simulink model "ev3_fix"  (R2018b)
settings: Solver=FixedStepAuto  StartTime=0.0  StopTime=10.0  RelTol=1e-3  EnableMultiTasking=on
libraries: legoev3lib x3
settings Model: ExtModeTrigDuration=2  Creator=chpark  LastModifiedBy=chpark
settings SolverCC: PositivePriorityOrder=on
settings OptimizationCC: EnhancedBackFolding=on  PassReuseOutputArgsAs=Individual arguments  MaxStackSize=64  OptimizeBlockOrder=speed  DifferentSizesBufferReuse=on  OptimizationCustomize=off
settings DebuggingCC: ParameterTunabilityLossMsg=error
settings HardwareCC: ProdBitPerPointer=32  ProdBitPerSizeT=32  ProdBitPerPtrDiffT=32  ProdLargestAtomicInteger=Long  ProdWordSize=32  ProdHWDeviceType=ARM Compatible->ARM 9  UseEmbeddedCoderFeatures=off  UseSimulinkCoderFeatures=off
settings SFSimCC: MATLABDynamicMemAlloc=off
settings RTWCC: SystemTargetFile=ert.tlc  HardwareBoard=LEGO MINDSTORMS EV3  TLCOptions="-aInlineSetEventsForThisBaseRateFcn=TLC_FALSE -aSuppressMultiTaskScheduler=TLC_FALSE  -aRateBasedStepFcn=0"  TemplateMakefile=ert_default_tmf  GenerateReport=on  Toolchain=Sourcery G++ Lite v2009q3  IncludeHyperlinkInReport=on  LaunchReport=on  GenerateTraceInfo=on  GenerateTraceReport=on  GenerateTraceReportSl=on  GenerateTraceReportSf=on  GenerateTraceReportEml=on
settings CodeAppCC: ForceParamTrailComments=on  IgnoreCustomStorageClasses=off  OperatorAnnotations=on  SimulinkDataObjDesc=on  SFDataObjDesc=on  InsertBlockDesc=on
settings ERTTargetCC: SupportContinuousTime=on  SupportNonInlinedSFcns=on  SupportVariableSizeSignals=on

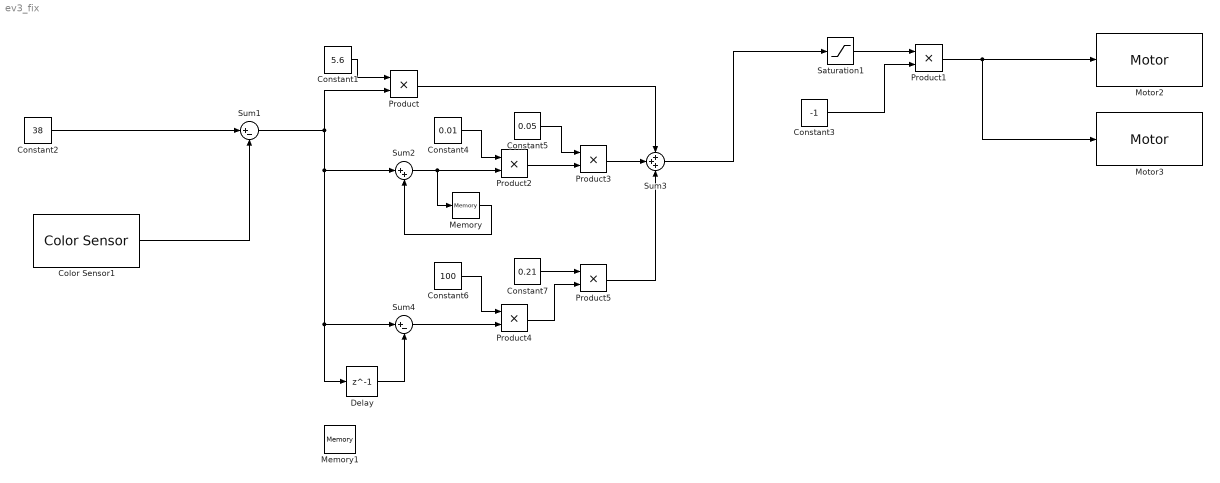
== system ev3_fix ==
  Color Sensor1 : legoev3lib/Color Sensor  portNumber=4  mode=Reflected light intensity  sampleTime=0.01
      settings: SourceProductName=Simulink Support Package for LEGO MINDSTORMS EV3 Hardware  SourceProductBaseCode=LEGOEV3
  Constant1 : Constant  Value=5.6
  Constant2 : Constant  Value=38
  Constant3 : Constant  Value=-1
  Constant4 : Constant  Value=0.01
  Constant5 : Constant  Value=0.05
  Constant6 : Constant  Value=100
  Constant7 : Constant  Value=0.21
  Delay : Delay  DelayLength=1  InitialCondition=0
  Memory : Memory
  Memory1 : Memory
  Motor2 : legoev3lib/Motor  sportNumber=A  sstopAction=Brake
  Motor3 : legoev3lib/Motor  sportNumber=D  sstopAction=Brake
  Product{,1..5} (6 alike) : Product
  Saturation1 : Saturate  UpperLimit=100  LowerLimit=-100
  Sum1 : Sum  Inputs=|+-
  Sum2 : Sum  Inputs=|++
  Sum3 : Sum  Inputs=+++
  Sum4 : Sum  Inputs=|+-
  wires:
  Constant2/1 -> Sum1/1
  Color Sensor1/1 -> Sum1/2
  Product1/1 -> Motor3/1, Motor2/1
  Saturation1/1 -> Product1/1
  Constant3/1 -> Product1/2
  Constant1/1 -> Product/1
  Sum1/1 -> Sum4/1, Delay/1, Sum2/1, Product/2
  Sum2/1 -> Product2/2, Memory/1
  Memory/1 -> Sum2/2
  Constant4/1 -> Product2/1
  Constant5/1 -> Product3/1
  Product2/1 -> Product3/2
  Product3/1 -> Sum3/2
  Product/1 -> Sum3/1
  Product5/1 -> Sum3/3
  Constant7/1 -> Product5/1
  Sum4/1 -> Product4/2
  Product4/1 -> Product5/2
  Constant6/1 -> Product4/1
  Sum3/1 -> Saturation1/1
  Delay/1 -> Sum4/2
